simulink model "Cascaded_Subsystem"  (R2020b)
settings: Solver=VariableStepAuto  StartTime=0.0  StopTime=10.0  RelTol=1e-3
settings Model: Creator=Hp  LastModifiedBy=Makrand Raut Dessai
settings DataIOCC: SaveOutput=off  SaveTime=off

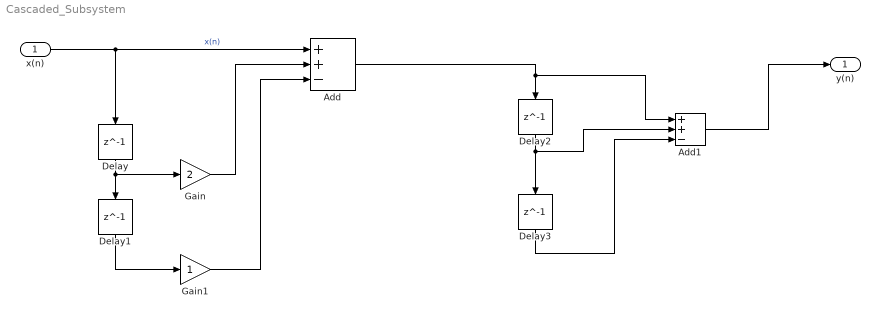
== system Cascaded_Subsystem ==
  x(n) : Inport  OutDataTypeStr=double  PortDimensions=1  SampleTime=[0,1]
  Add : Sum  Inputs=++-
  Add1 : Sum  Inputs=++-
  Delay{,1..3} (4 alike) : Delay  DelayLength=1
  Gain : Gain  Gain=2
  Gain1 : Gain
  y(n) : Outport  OutDataTypeStr=double  PortDimensions=1  SampleTime=[0,1]
  wires:
  x(n)/1 -> Add/1, Delay/1  "x(n)"
  Delay/1 -> Delay1/1, Gain/1
  Gain/1 -> Add/2
  Gain1/1 -> Add/3
  Delay1/1 -> Gain1/1
  Add/1 -> Add1/1, Delay2/1
  Delay2/1 -> Add1/2, Delay3/1
  Delay3/1 -> Add1/3
  Add1/1 -> y(n)/1
